simulink model "ControlPendulo2GDL_PNL"  (R2019b)
settings: Solver=ode45  StartTime=0.0  StopTime=ts  FixedStep=0.01  RelTol=1e-3
values from neighbouring files (symbols this model uses):
  b1 = c8    (= 0.01)    [PenduloDatos.m]
  b2 = c8    (= 0.01)    [PenduloDatos.m]
  C = [1 0 0 0]    [PenduloDatos.m]
  g = 9.78    [PenduloDatos.m]
  I1 = 1/12*m1*(a1^2+d1^2)    (= 3.14166666667e-05)    [PenduloDatos.m]
  I2 = 1/12*m2*(a2^2+d2^2)    (= 1.20833333333e-05)    [PenduloDatos.m]
  K = place(Al,Bl,[Pd1 Pd2 Pd3 Pd4])    [PenduloDatos.m]
  K0 = inv(C*(inv(-Al+Bl*K))*Bl)    [PenduloDatos.m]
  K0D = inv(CD*inv(eye(4)-AD+BD*KD)*BD)    [PenduloDatos.m]
  KD = place(AD,BD,exp([Pd1 Pd2 Pd3 Pd4]*tm))    [PenduloDatos.m]
  L = place(Al',C',[5*Pd1 5*Pd2 5*Pd3 5*Pd4])'    [PenduloDatos.m]
  l1 = c1    (= 0.3)    [PenduloDatos.m]
  l2 = c2    (= 0.2)    [PenduloDatos.m]
  lc1 = 0.25    [PenduloDatos.m]
  lc2 = 0.11    [PenduloDatos.m]
  LD = place(AD',CD',exp([5*Pd1 5*Pd2 5*Pd3 5*Pd4]*tm))'    [PenduloDatos.m]
  m1 = c3    (= 0.065)    [PenduloDatos.m]
  m2 = c4    (= 0.025)    [PenduloDatos.m]
  Ref = 0.2    [PenduloDatos.m]
  tm = 0.01    [PenduloDatos.m]
  U0 = [Tau1]    [PenduloDatos.m]
  X0 = [Tt1;Tpt1;Tt2;Tpt2]    [PenduloDatos.m]
  XI = [0;0;0;0]    [PenduloDatos.m]
undefined symbols (not defined in the file or in its folder): AD, Al, BD, Bl, CD
libraries: simulink x4
settings Model: Creator=ARQ SEVILLA R  LastModifiedBy=ARQ SEVILLA R

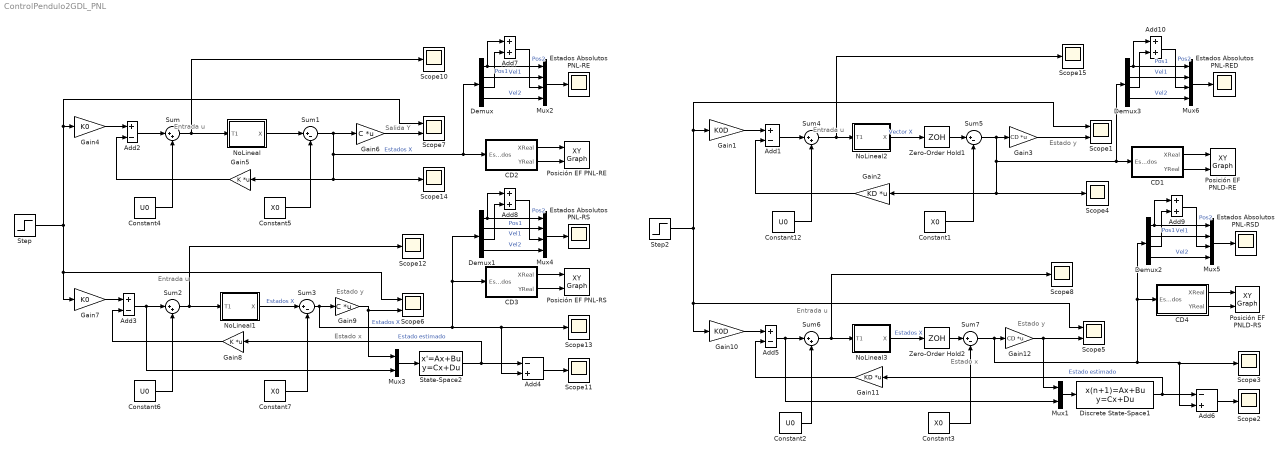
== system ControlPendulo2GDL_PNL ==
  note: Salida Y
  note: Entrada u
  note: Entrada u
  note: Estado y
  note: Estado x
  note: Estado y
  note: Entrada u
  note: Estado x
  note: Entrada u
  note: Estado y
  Add{1..3,5} (4 alike) : Sum  Inputs=+-
  Add{7..10} (4 alike) : Sum
  Add4 : Sum  Inputs=-+
  Add6 : Sum  Inputs=-+
  CD1 : Subsystem  TreatAsAtomicUnit=on
  CD2 : Subsystem  TreatAsAtomicUnit=on
  CD3 : Subsystem  TreatAsAtomicUnit=on
  CD4 : Subsystem  TreatAsAtomicUnit=on
  Constant{1,3,5,7} (4 alike) : Constant  Value=X0
  Constant{2,4,6,12} (4 alike) : Constant  Value=U0
  Demux{,1..3} (4 alike) : Demux
  Discrete State-Space1 : DiscreteStateSpace  A=AD-LD*CD  B=[LD BD]  C=eye(4)  D=zeros(4,2)  InitialCondition=XI  SampleTime=tm
  Estados Absolutos PNL-RE : Scope
  Estados Absolutos PNL-RED : Scope
  Estados Absolutos PNL-RS : Scope
  Estados Absolutos PNL-RSD : Scope
  Gain1 : Gain  Gain=K0D
  Gain10 : Gain  Gain=K0D
  Gain11 : Gain  Gain=KD  Multiplication=Matrix(K*u)
  Gain12 : Gain  Gain=CD  Multiplication=Matrix(K*u)
  Gain2 : Gain  Gain=KD  Multiplication=Matrix(K*u)
  Gain3 : Gain  Gain=CD  Multiplication=Matrix(K*u)
  Gain4 : Gain  Gain=K0
  Gain5 : Gain  Gain=K  Multiplication=Matrix(K*u)
  Gain6 : Gain  Gain=C  Multiplication=Matrix(K*u)
  Gain7 : Gain  Gain=K0
  Gain8 : Gain  Gain=K  Multiplication=Matrix(K*u)
  Gain9 : Gain  Gain=C  Multiplication=Matrix(K*u)
  Mux1 : Mux  Inputs=2
  Mux{2,4..6} (4 alike) : Mux
  Mux3 : Mux  Inputs=2
  NoLineal : Subsystem
  NoLineal1 : Subsystem
  NoLineal2 : Subsystem
  NoLineal3 : Subsystem
  Posición EF PNL-RE : simulink/Sinks/XY Graph  xmin=-l2-l1  xmax=l2+l1  ymin=-l2-l1  ymax=l2+l1  st=-1
  Posición EF PNL-RS : simulink/Sinks/XY Graph  xmin=-l2-l1  xmax=l2+l1  ymin=-l2-l1  ymax=l2+l1  st=-1
  Posición EF PNLD-RE : simulink/Sinks/XY Graph  xmin=-l2-l1  xmax=l2+l1  ymin=-l2-l1  ymax=l2+l1  st=-1
  Posición EF PNLD-RS : simulink/Sinks/XY Graph  xmin=-l2-l1  xmax=l2+l1  ymin=-l2-l1  ymax=l2+l1  st=-1
  Scope{1,5..7} (4 alike) : Scope  NumInputPorts=2
  Scope{2..4,8,10..15} (10 alike) : Scope
  State-Space2 : StateSpace  A=Al-L*C  B=[L,Bl]  C=eye(4)  D=zeros(4,2)  InitialCondition=XI
  Step : Step  Time=0  After=Ref  SampleTime=0
  Step2 : Step  Time=0  After=Ref  SampleTime=tm
  Sum{,2,4,6} (4 alike) : Sum  Inputs=|++
  Sum{1,3,5,7} (4 alike) : Sum  Inputs=|+-
  Zero-Order Hold1 : ZeroOrderHold  SampleTime=tm
  Zero-Order Hold2 : ZeroOrderHold  SampleTime=tm
  wires:
  Add2/1 -> Sum/1
  Sum/1 -> NoLineal/1(T1), Scope10/1
  Sum2/1 -> NoLineal1/1(T1), Scope12/1
  Constant5/1 -> Sum1/2
  Add4/1 -> Scope11/1
  Constant4/1 -> Sum/2
  State-Space2/1 -> Add4/1, Gain8/1  "Estado estimado"
  Constant7/1 -> Sum3/2
  Add3/1 -> Mux3/2, Sum2/1
  Gain7/1 -> Add3/1
  Gain8/1 -> Add3/2
  Constant6/1 -> Sum2/2
  Gain9/1 -> Scope6/2, Mux3/1
  Gain4/1 -> Add2/1
  Mux3/1 -> State-Space2/1
  Gain5/1 -> Add2/2
  Gain6/1 -> Scope7/2
  CD2/2(YReal) -> Posición EF PNL-RE/2
  CD2/1(XReal) -> Posición EF PNL-RE/1
  CD3/1(XReal) -> Posición EF PNL-RS/1
  CD3/2(YReal) -> Posición EF PNL-RS/2
  NoLineal1/1(X) -> Sum3/1  "Estados X"
  Add1/1 -> Sum4/1
  Constant1/1 -> Sum5/2
  Constant12/1 -> Sum4/2
  Constant3/1 -> Sum7/2
  Gain11/1 -> Add5/2
  Sum4/1 -> NoLineal2/1(T1), Scope15/1
  Gain1/1 -> Add1/1
  Sum7/1 -> Demux2/1, CD4/1(Estados), Scope3/1, Add6/2, Gain12/1
  NoLineal2/1(X) -> Zero-Order Hold1/1  "Vector X"
  Gain2/1 -> Add1/2
  Gain12/1 -> Scope5/2, Mux1/1
  Sum6/1 -> NoLineal3/1(T1), Scope8/1
  Constant2/1 -> Sum6/2
  Add5/1 -> Mux1/2, Sum6/1
  Mux1/1 -> Discrete State-Space1/1
  Discrete State-Space1/1 -> Add6/1, Gain11/1  "Estado estimado"
  Gain3/1 -> Scope1/2
  Gain10/1 -> Add5/1
  Add6/1 -> Scope2/1
  Zero-Order Hold1/1 -> Sum5/1
  Zero-Order Hold2/1 -> Sum7/1
  CD1/1(XReal) -> Posición EF PNLD-RE/1
  CD1/2(YReal) -> Posición EF PNLD-RE/2
  CD4/2(YReal) -> Posición EF PNLD-RS/2
  CD4/1(XReal) -> Posición EF PNLD-RS/1
  NoLineal/1(X) -> Sum1/1
  NoLineal3/1(X) -> Zero-Order Hold2/1  "Estados X"
  Demux/4 -> Mux2/4  "Vel2"
  Demux/2 -> Mux2/2  "Vel1"
  Add7/1 -> Mux2/3  "Pos2"
  Sum1/1 -> Demux/1, CD2/1(Estados), Scope14/1, Gain5/1, Gain6/1  "Estados X"
  Mux2/1 -> Estados Absolutos PNL-RE/1
  Demux/1 -> Add7/1, Mux2/1  "Pos1"
  Demux/3 -> Add7/2
  Demux1/3 -> Add8/2
  Demux1/1 -> Mux4/1, Add8/1  "Pos1"
  Mux4/1 -> Estados Absolutos PNL-RS/1
  Sum3/1 -> Demux1/1, CD3/1(Estados), Scope13/1, Add4/2, Gain9/1  "Estados X"
  Add8/1 -> Mux4/3  "Pos2"
  Demux1/2 -> Mux4/2  "Vel1"
  Demux1/4 -> Mux4/4  "Vel2"
  Demux2/4 -> Mux5/4  "Vel2"
  Demux2/2 -> Mux5/2  "Vel1"
  Add9/1 -> Mux5/3  "Pos2"
  Mux5/1 -> Estados Absolutos PNL-RSD/1
  Demux2/1 -> Add9/1, Mux5/1  "Pos1"
  Demux2/3 -> Add9/2
  Demux3/3 -> Add10/2
  Demux3/1 -> Mux6/1, Add10/1  "Pos1"
  Mux6/1 -> Estados Absolutos PNL-RED/1
  Add10/1 -> Mux6/3  "Pos2"
  Demux3/2 -> Mux6/2  "Vel1"
  Demux3/4 -> Mux6/4  "Vel2"
  Sum5/1 -> Demux3/1, CD1/1(Estados), Scope4/1, Gain2/1, Gain3/1
  Step/1 -> Scope6/1, Gain7/1, Scope7/1, Gain4/1
  Step2/1 -> Scope1/1, Gain1/1, Scope5/1, Gain10/1

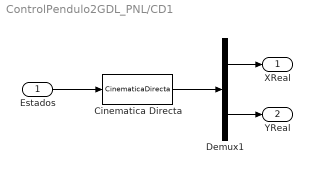
== system ControlPendulo2GDL_PNL/CD1 ==
  Estados : Inport
  Cinematica Directa : MATLABFcn  MATLABFcn=CinematicaDirecta  OutputDimensions=2
  Demux1 : Demux  Outputs=2
  XReal : Outport  VectorParamsAs1DForOutWhenUnconnected=off
  YReal : Outport  Port=2  VectorParamsAs1DForOutWhenUnconnected=off
  wires:
  Estados/1 -> Cinematica Directa/1
  Demux1/2 -> YReal/1
  Demux1/1 -> XReal/1
  Cinematica Directa/1 -> Demux1/1

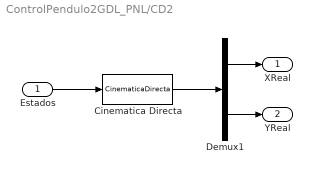
== system ControlPendulo2GDL_PNL/CD2 ==
  Estados : Inport
  Cinematica Directa : MATLABFcn  MATLABFcn=CinematicaDirecta  OutputDimensions=2
  Demux1 : Demux  Outputs=2
  XReal : Outport  VectorParamsAs1DForOutWhenUnconnected=off
  YReal : Outport  Port=2  VectorParamsAs1DForOutWhenUnconnected=off
  wires:
  Cinematica Directa/1 -> Demux1/1
  Demux1/1 -> XReal/1
  Demux1/2 -> YReal/1
  Estados/1 -> Cinematica Directa/1

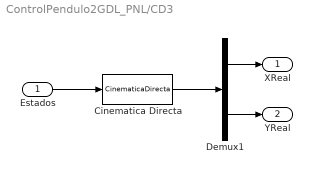
== system ControlPendulo2GDL_PNL/CD3 ==
  Estados : Inport
  Cinematica Directa : MATLABFcn  MATLABFcn=CinematicaDirecta  OutputDimensions=2
  Demux1 : Demux  Outputs=2
  XReal : Outport  VectorParamsAs1DForOutWhenUnconnected=off
  YReal : Outport  Port=2  VectorParamsAs1DForOutWhenUnconnected=off
  wires:
  Estados/1 -> Cinematica Directa/1
  Demux1/2 -> YReal/1
  Demux1/1 -> XReal/1
  Cinematica Directa/1 -> Demux1/1

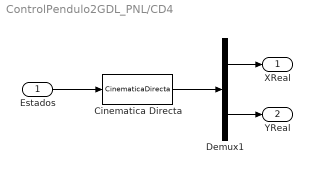
== system ControlPendulo2GDL_PNL/CD4 ==
  Estados : Inport
  Cinematica Directa : MATLABFcn  MATLABFcn=CinematicaDirecta  OutputDimensions=2
  Demux1 : Demux  Outputs=2
  XReal : Outport  VectorParamsAs1DForOutWhenUnconnected=off
  YReal : Outport  Port=2  VectorParamsAs1DForOutWhenUnconnected=off
  wires:
  Cinematica Directa/1 -> Demux1/1
  Demux1/1 -> XReal/1
  Demux1/2 -> YReal/1
  Estados/1 -> Cinematica Directa/1

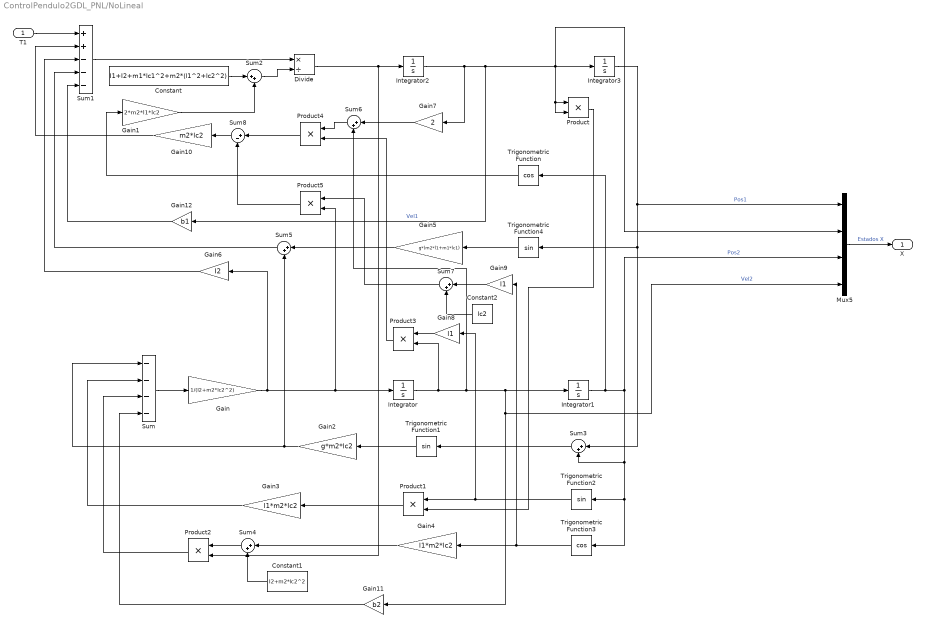
== system ControlPendulo2GDL_PNL/NoLineal ==
  T1 : Inport
  Constant : Constant  Value=I1+I2+m1*lc1^2+m2*(l1^2+lc2^2)
  Constant1 : Constant  Value=I2+m2*lc2^2
  Constant2 : Constant  Value=lc2
  Divide : Product  Inputs=*/
  Gain : Gain  Gain=1/(I2+m2*lc2^2)
  Gain1 : Gain  Gain=2*m2*l1*lc2
  Gain10 : Gain  Gain=m2*lc2
  Gain11 : Gain  Gain=b2
  Gain12 : Gain  Gain=b1
  Gain2 : Gain  Gain=g*m2*lc2
  Gain3 : Gain  Gain=l1*m2*lc2
  Gain4 : Gain  Gain=l1*m2*lc2
  Gain5 : Gain  Gain=g*(m2*l1+m1*lc1)
  Gain6 : Gain  Gain=I2
  Gain7 : Gain  Gain=2
  Gain8 : Gain  Gain=l1
  Gain9 : Gain  Gain=l1
  Integrator : Integrator  InitialCondition=X0(4)
  Integrator1 : Integrator  InitialCondition=X0(3)
  Integrator2 : Integrator  InitialCondition=X0(2)
  Integrator3 : Integrator  InitialCondition=X0(1)
  Mux5 : Mux
  Product{,1..5} (6 alike) : Product
  Sum : Sum  Inputs=----
  Sum1 : Sum  Inputs=++---
  Sum{2..7} (6 alike) : Sum  Inputs=|++
  Sum8 : Sum  Inputs=|+-
  Trigonometric Function : Trigonometry  Operator=cos
  Trigonometric Function1 : Trigonometry
  Trigonometric Function2 : Trigonometry
  Trigonometric Function3 : Trigonometry  Operator=cos
  Trigonometric Function4 : Trigonometry
  X : Outport  VectorParamsAs1DForOutWhenUnconnected=off
  wires:
  Integrator/1 -> Product3/2, Gain11/1, Mux5/4, Integrator1/1, Sum6/2  "Vel2"
  Product4/1 -> Sum8/1
  Gain10/1 -> Sum1/2
  Constant/1 -> Sum2/1
  Sum7/1 -> Product5/1
  Sum1/1 -> Divide/1
  Gain6/1 -> Sum1/3
  Integrator1/1 -> Trigonometric Function/1, Mux5/3, Trigonometric Function3/1, Trigonometric Function2/1, Sum3/2  "Pos2"
  Sum3/1 -> Trigonometric Function1/1
  Gain11/1 -> Sum/4
  Product/1 -> Product1/2
  Gain4/1 -> Sum4/1
  Sum/1 -> Gain/1
  Constant2/1 -> Sum7/2
  Gain8/1 -> Product3/1
  Trigonometric Function3/1 -> Gain9/1, Gain4/1
  Product1/1 -> Gain3/1
  Gain7/1 -> Sum6/1
  Trigonometric Function2/1 -> Gain8/1, Product1/1
  Sum8/1 -> Gain10/1
  Gain2/1 -> Sum5/2, Sum/1
  Constant1/1 -> Sum4/2
  Integrator2/1 -> Gain7/1, Integrator3/1, Mux5/2, Product/2, Product/1, Gain12/1  "Vel1"
  Trigonometric Function4/1 -> Gain5/1
  Divide/1 -> Product2/2, Integrator2/1
  Product5/1 -> Sum8/2
  Gain3/1 -> Sum/2
  Gain9/1 -> Sum7/1
  T1/1 -> Sum1/1
  Gain/1 -> Product5/2, Integrator/1, Gain6/1
  Product3/1 -> Product4/2
  Sum2/1 -> Divide/2
  Sum6/1 -> Product4/1
  Integrator3/1 -> Mux5/1, Sum3/1, Trigonometric Function4/1  "Pos1"
  Trigonometric Function/1 -> Gain1/1
  Gain1/1 -> Sum2/2
  Sum5/1 -> Sum1/4
  Gain5/1 -> Sum5/1
  Gain12/1 -> Sum1/5
  Product2/1 -> Sum/3
  Sum4/1 -> Product2/1
  Trigonometric Function1/1 -> Gain2/1
  Mux5/1 -> X/1  "Estados X"

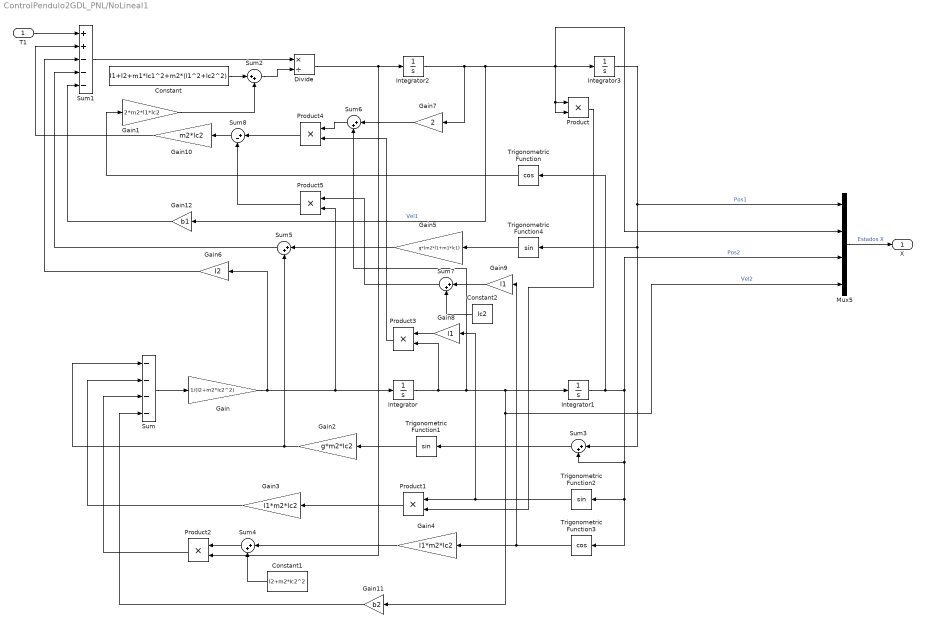
== system ControlPendulo2GDL_PNL/NoLineal1 ==
  T1 : Inport
  Constant : Constant  Value=I1+I2+m1*lc1^2+m2*(l1^2+lc2^2)
  Constant1 : Constant  Value=I2+m2*lc2^2
  Constant2 : Constant  Value=lc2
  Divide : Product  Inputs=*/
  Gain : Gain  Gain=1/(I2+m2*lc2^2)
  Gain1 : Gain  Gain=2*m2*l1*lc2
  Gain10 : Gain  Gain=m2*lc2
  Gain11 : Gain  Gain=b2
  Gain12 : Gain  Gain=b1
  Gain2 : Gain  Gain=g*m2*lc2
  Gain3 : Gain  Gain=l1*m2*lc2
  Gain4 : Gain  Gain=l1*m2*lc2
  Gain5 : Gain  Gain=g*(m2*l1+m1*lc1)
  Gain6 : Gain  Gain=I2
  Gain7 : Gain  Gain=2
  Gain8 : Gain  Gain=l1
  Gain9 : Gain  Gain=l1
  Integrator : Integrator  InitialCondition=X0(4)
  Integrator1 : Integrator  InitialCondition=X0(3)
  Integrator2 : Integrator  InitialCondition=X0(2)
  Integrator3 : Integrator  InitialCondition=X0(1)
  Mux5 : Mux
  Product{,1..5} (6 alike) : Product
  Sum : Sum  Inputs=----
  Sum1 : Sum  Inputs=++---
  Sum{2..7} (6 alike) : Sum  Inputs=|++
  Sum8 : Sum  Inputs=|+-
  Trigonometric Function : Trigonometry  Operator=cos
  Trigonometric Function1 : Trigonometry
  Trigonometric Function2 : Trigonometry
  Trigonometric Function3 : Trigonometry  Operator=cos
  Trigonometric Function4 : Trigonometry
  X : Outport  VectorParamsAs1DForOutWhenUnconnected=off
  wires:
  Integrator/1 -> Product3/2, Gain11/1, Mux5/4, Integrator1/1, Sum6/2  "Vel2"
  Product4/1 -> Sum8/1
  Gain10/1 -> Sum1/2
  Constant/1 -> Sum2/1
  Sum7/1 -> Product5/1
  Sum1/1 -> Divide/1
  Gain6/1 -> Sum1/3
  Integrator1/1 -> Trigonometric Function/1, Mux5/3, Trigonometric Function3/1, Trigonometric Function2/1, Sum3/2  "Pos2"
  Sum3/1 -> Trigonometric Function1/1
  Gain11/1 -> Sum/4
  Product/1 -> Product1/2
  Gain4/1 -> Sum4/1
  Sum/1 -> Gain/1
  Constant2/1 -> Sum7/2
  Gain8/1 -> Product3/1
  Trigonometric Function3/1 -> Gain9/1, Gain4/1
  Product1/1 -> Gain3/1
  Gain7/1 -> Sum6/1
  Trigonometric Function2/1 -> Gain8/1, Product1/1
  Sum8/1 -> Gain10/1
  Gain2/1 -> Sum5/2, Sum/1
  Constant1/1 -> Sum4/2
  Integrator2/1 -> Gain7/1, Integrator3/1, Mux5/2, Product/2, Product/1, Gain12/1  "Vel1"
  Trigonometric Function4/1 -> Gain5/1
  Divide/1 -> Product2/2, Integrator2/1
  Product5/1 -> Sum8/2
  Gain3/1 -> Sum/2
  Gain9/1 -> Sum7/1
  T1/1 -> Sum1/1
  Gain/1 -> Product5/2, Integrator/1, Gain6/1
  Product3/1 -> Product4/2
  Sum2/1 -> Divide/2
  Sum6/1 -> Product4/1
  Integrator3/1 -> Mux5/1, Sum3/1, Trigonometric Function4/1  "Pos1"
  Trigonometric Function/1 -> Gain1/1
  Gain1/1 -> Sum2/2
  Sum5/1 -> Sum1/4
  Gain5/1 -> Sum5/1
  Gain12/1 -> Sum1/5
  Product2/1 -> Sum/3
  Sum4/1 -> Product2/1
  Trigonometric Function1/1 -> Gain2/1
  Mux5/1 -> X/1  "Estados X"

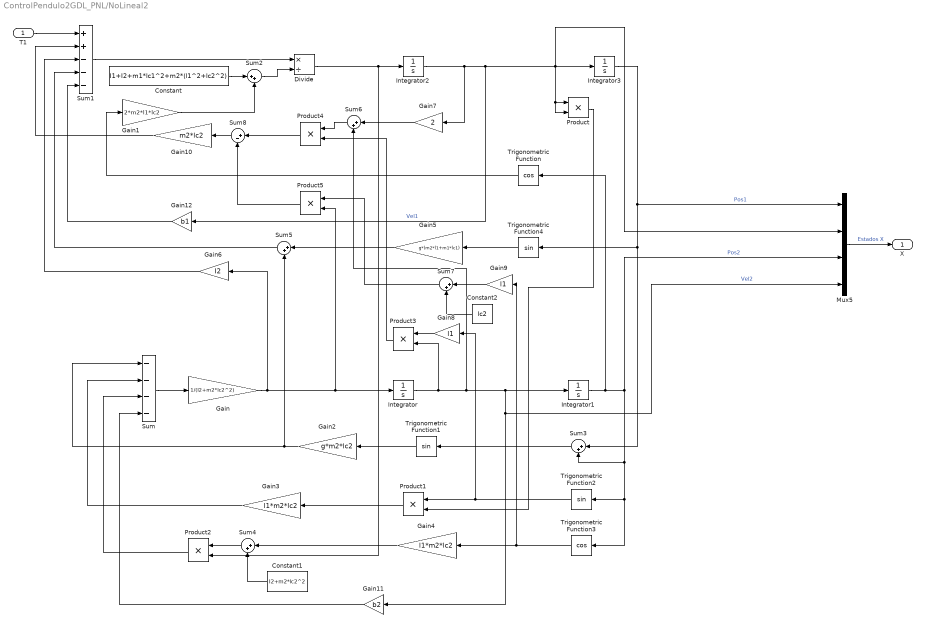
== system ControlPendulo2GDL_PNL/NoLineal2 ==
  T1 : Inport
  Constant : Constant  Value=I1+I2+m1*lc1^2+m2*(l1^2+lc2^2)
  Constant1 : Constant  Value=I2+m2*lc2^2
  Constant2 : Constant  Value=lc2
  Divide : Product  Inputs=*/
  Gain : Gain  Gain=1/(I2+m2*lc2^2)
  Gain1 : Gain  Gain=2*m2*l1*lc2
  Gain10 : Gain  Gain=m2*lc2
  Gain11 : Gain  Gain=b2
  Gain12 : Gain  Gain=b1
  Gain2 : Gain  Gain=g*m2*lc2
  Gain3 : Gain  Gain=l1*m2*lc2
  Gain4 : Gain  Gain=l1*m2*lc2
  Gain5 : Gain  Gain=g*(m2*l1+m1*lc1)
  Gain6 : Gain  Gain=I2
  Gain7 : Gain  Gain=2
  Gain8 : Gain  Gain=l1
  Gain9 : Gain  Gain=l1
  Integrator : Integrator  InitialCondition=X0(4)
  Integrator1 : Integrator  InitialCondition=X0(3)
  Integrator2 : Integrator  InitialCondition=X0(2)
  Integrator3 : Integrator  InitialCondition=X0(1)
  Mux5 : Mux
  Product{,1..5} (6 alike) : Product
  Sum : Sum  Inputs=----
  Sum1 : Sum  Inputs=++---
  Sum{2..7} (6 alike) : Sum  Inputs=|++
  Sum8 : Sum  Inputs=|+-
  Trigonometric Function : Trigonometry  Operator=cos
  Trigonometric Function1 : Trigonometry
  Trigonometric Function2 : Trigonometry
  Trigonometric Function3 : Trigonometry  Operator=cos
  Trigonometric Function4 : Trigonometry
  X : Outport  VectorParamsAs1DForOutWhenUnconnected=off
  wires:
  Integrator/1 -> Product3/2, Gain11/1, Mux5/4, Integrator1/1, Sum6/2  "Vel2"
  Product4/1 -> Sum8/1
  Gain10/1 -> Sum1/2
  Constant/1 -> Sum2/1
  Sum7/1 -> Product5/1
  Sum1/1 -> Divide/1
  Gain6/1 -> Sum1/3
  Integrator1/1 -> Trigonometric Function/1, Mux5/3, Trigonometric Function3/1, Trigonometric Function2/1, Sum3/2  "Pos2"
  Sum3/1 -> Trigonometric Function1/1
  Gain11/1 -> Sum/4
  Product/1 -> Product1/2
  Gain4/1 -> Sum4/1
  Sum/1 -> Gain/1
  Constant2/1 -> Sum7/2
  Gain8/1 -> Product3/1
  Trigonometric Function3/1 -> Gain9/1, Gain4/1
  Product1/1 -> Gain3/1
  Gain7/1 -> Sum6/1
  Trigonometric Function2/1 -> Gain8/1, Product1/1
  Sum8/1 -> Gain10/1
  Gain2/1 -> Sum5/2, Sum/1
  Constant1/1 -> Sum4/2
  Integrator2/1 -> Gain7/1, Integrator3/1, Mux5/2, Product/2, Product/1, Gain12/1  "Vel1"
  Trigonometric Function4/1 -> Gain5/1
  Divide/1 -> Product2/2, Integrator2/1
  Product5/1 -> Sum8/2
  Gain3/1 -> Sum/2
  Gain9/1 -> Sum7/1
  T1/1 -> Sum1/1
  Gain/1 -> Product5/2, Integrator/1, Gain6/1
  Product3/1 -> Product4/2
  Sum2/1 -> Divide/2
  Sum6/1 -> Product4/1
  Integrator3/1 -> Mux5/1, Sum3/1, Trigonometric Function4/1  "Pos1"
  Trigonometric Function/1 -> Gain1/1
  Gain1/1 -> Sum2/2
  Sum5/1 -> Sum1/4
  Gain5/1 -> Sum5/1
  Gain12/1 -> Sum1/5
  Product2/1 -> Sum/3
  Sum4/1 -> Product2/1
  Trigonometric Function1/1 -> Gain2/1
  Mux5/1 -> X/1  "Estados X"

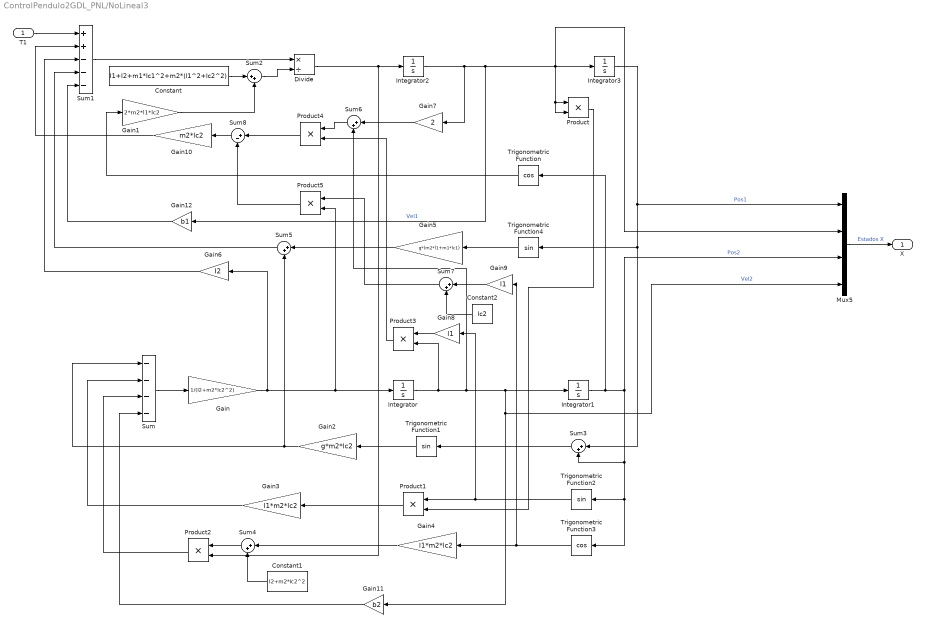
== system ControlPendulo2GDL_PNL/NoLineal3 ==
  T1 : Inport
  Constant : Constant  Value=I1+I2+m1*lc1^2+m2*(l1^2+lc2^2)
  Constant1 : Constant  Value=I2+m2*lc2^2
  Constant2 : Constant  Value=lc2
  Divide : Product  Inputs=*/
  Gain : Gain  Gain=1/(I2+m2*lc2^2)
  Gain1 : Gain  Gain=2*m2*l1*lc2
  Gain10 : Gain  Gain=m2*lc2
  Gain11 : Gain  Gain=b2
  Gain12 : Gain  Gain=b1
  Gain2 : Gain  Gain=g*m2*lc2
  Gain3 : Gain  Gain=l1*m2*lc2
  Gain4 : Gain  Gain=l1*m2*lc2
  Gain5 : Gain  Gain=g*(m2*l1+m1*lc1)
  Gain6 : Gain  Gain=I2
  Gain7 : Gain  Gain=2
  Gain8 : Gain  Gain=l1
  Gain9 : Gain  Gain=l1
  Integrator : Integrator  InitialCondition=X0(4)
  Integrator1 : Integrator  InitialCondition=X0(3)
  Integrator2 : Integrator  InitialCondition=X0(2)
  Integrator3 : Integrator  InitialCondition=X0(1)
  Mux5 : Mux
  Product{,1..5} (6 alike) : Product
  Sum : Sum  Inputs=----
  Sum1 : Sum  Inputs=++---
  Sum{2..7} (6 alike) : Sum  Inputs=|++
  Sum8 : Sum  Inputs=|+-
  Trigonometric Function : Trigonometry  Operator=cos
  Trigonometric Function1 : Trigonometry
  Trigonometric Function2 : Trigonometry
  Trigonometric Function3 : Trigonometry  Operator=cos
  Trigonometric Function4 : Trigonometry
  X : Outport  VectorParamsAs1DForOutWhenUnconnected=off
  wires:
  Integrator/1 -> Product3/2, Gain11/1, Mux5/4, Integrator1/1, Sum6/2  "Vel2"
  Product4/1 -> Sum8/1
  Gain10/1 -> Sum1/2
  Constant/1 -> Sum2/1
  Sum7/1 -> Product5/1
  Sum1/1 -> Divide/1
  Gain6/1 -> Sum1/3
  Integrator1/1 -> Trigonometric Function/1, Mux5/3, Trigonometric Function3/1, Trigonometric Function2/1, Sum3/2  "Pos2"
  Sum3/1 -> Trigonometric Function1/1
  Gain11/1 -> Sum/4
  Product/1 -> Product1/2
  Gain4/1 -> Sum4/1
  Sum/1 -> Gain/1
  Constant2/1 -> Sum7/2
  Gain8/1 -> Product3/1
  Trigonometric Function3/1 -> Gain9/1, Gain4/1
  Product1/1 -> Gain3/1
  Gain7/1 -> Sum6/1
  Trigonometric Function2/1 -> Gain8/1, Product1/1
  Sum8/1 -> Gain10/1
  Gain2/1 -> Sum5/2, Sum/1
  Constant1/1 -> Sum4/2
  Integrator2/1 -> Gain7/1, Integrator3/1, Mux5/2, Product/2, Product/1, Gain12/1  "Vel1"
  Trigonometric Function4/1 -> Gain5/1
  Divide/1 -> Product2/2, Integrator2/1
  Product5/1 -> Sum8/2
  Gain3/1 -> Sum/2
  Gain9/1 -> Sum7/1
  T1/1 -> Sum1/1
  Gain/1 -> Product5/2, Integrator/1, Gain6/1
  Product3/1 -> Product4/2
  Sum2/1 -> Divide/2
  Sum6/1 -> Product4/1
  Integrator3/1 -> Mux5/1, Sum3/1, Trigonometric Function4/1  "Pos1"
  Trigonometric Function/1 -> Gain1/1
  Gain1/1 -> Sum2/2
  Sum5/1 -> Sum1/4
  Gain5/1 -> Sum5/1
  Gain12/1 -> Sum1/5
  Product2/1 -> Sum/3
  Sum4/1 -> Product2/1
  Trigonometric Function1/1 -> Gain2/1
  Mux5/1 -> X/1  "Estados X"
